simulink library "inp_lib"  (Simulink 7.4)
settings: Solver=ode45  StartTime=0.0  StopTime=10.0  RelTol=1e-3
settings Model: Creator=gephn  LastModifiedBy=wuqnj

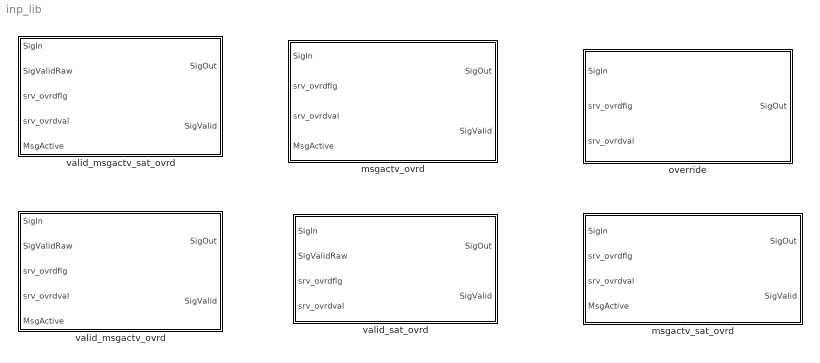
== system inp_lib ==
  msgactv_ovrd : Subsystem  mask{cal_ovrdflg=0, cal_ovrdval=0, default=0}
      mask prompts: cal_ovrdflg "Override Flag"; cal_ovrdval "Override Value"; default "Default Value"
  msgactv_sat_ovrd : Subsystem  mask{cal_ovrdflg=0, cal_ovrdval=0, default=0, hi=0, lo=0}
      mask prompts: cal_ovrdflg "Override Flag"; cal_ovrdval "Override Value"; default "Default Value"; hi "Range High"; lo "Range Low"
  override : Subsystem  mask{cal_ovrdflg=0, cal_ovrdval=0}
      mask prompts: cal_ovrdflg "Override Flag"; cal_ovrdval "Override Value"
  valid_msgactv_ovrd : Subsystem  AncestorBlock=inp_lib/valid_msgactv_sat_ovrd  mask{cal_ovrdflg=0, cal_ovrdval=0, lim=1, inc=1, dec=1, default=0}
      mask prompts: cal_ovrdflg "Override Flag"; cal_ovrdval "Override Value"; lim "Debounce Limit"; inc "Debounce Increment"; dec "Debounce Decrement"; default "Default Value"
  valid_msgactv_sat_ovrd : Subsystem  mask{cal_ovrdflg=0, cal_ovrdval=0, lim=1, inc=1, dec=1, default=0, hi=1, lo=0}
      mask prompts: cal_ovrdflg "Override Flag"; cal_ovrdval "Override Value"; lim "Debounce Limit"; inc "Debounce Increment"; dec "Debounce Decrement"; default "Default Value"; hi "Range High"; lo "Range Low"
  valid_sat_ovrd : Subsystem  mask{cal_ovrdflg=0, cal_ovrdval=0, lim=1, inc=1, dec=1, default=0, hi=1, lo=0}
      mask prompts: cal_ovrdflg "Override Flag"; cal_ovrdval "Override Value"; lim "Debounce Limit"; inc "Debounce Increment"; dec "Debounce Decrement"; default "Default Value"; hi "Range High"; lo "Range Low"

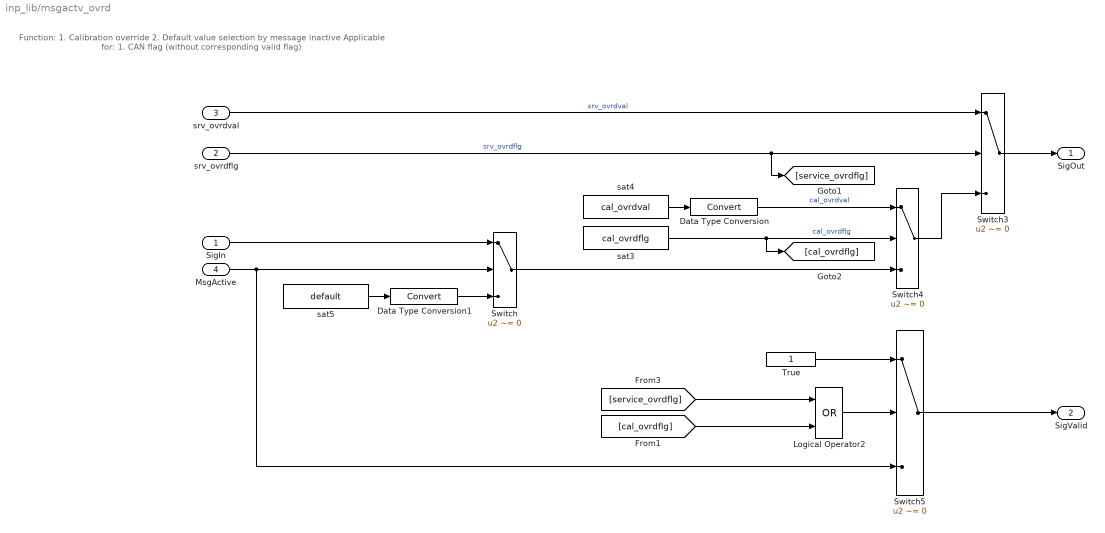
== system inp_lib/msgactv_ovrd ==
  note: Function:
      | 1. Calibration override
      | 2. Default value selection by message inactive
      | Applicable for:
      | 1. CAN flag  (without corresponding valid flag)
  SigIn : Inport  OutDataType=fixdt(1, 16)  OutScaling=2^0
  srv_ovrdflg : Inport  Port=2  OutDataType=fixdt(1, 16)  OutScaling=2^0
  srv_ovrdval : Inport  Port=3  OutDataType=fixdt(1, 16)  OutScaling=2^0
  MsgActive : Inport  Port=4  OutDataType=fixdt(1, 16)  OutScaling=2^0
  Data Type Conversion : DataTypeConversion  OutDataType=fixdt(1, 16)  OutScaling=2^0
  Data Type Conversion1 : DataTypeConversion  OutDataType=fixdt(1, 16)  OutScaling=2^0
  Logical Operator2 : Logic  Operator=OR  AllPortsSameDT=off  OutDataTypeMode=boolean  OutDataTypeStr=boolean
  Switch : Switch  Criteria=u2 ~= 0  OutDataType=fixdt(1, 16)  OutScaling=2^0
  Switch3 : Switch  Criteria=u2 ~= 0  Threshold=0.5  OutDataType=sfix(16)  OutScaling=2^0
  Switch4 : Switch  Criteria=u2 ~= 0  Threshold=0.5  OutDataType=sfix(16)  OutScaling=2^0
  Switch5 : Switch  Criteria=u2 ~= 0  Threshold=0.5  OutDataType=sfix(16)  OutScaling=2^0
  True : Constant  OutDataTypeMode=boolean  OutDataType=sfix(16)  OutScaling=2^0  OutDataTypeStr=boolean
  sat3 : Constant  Value=cal_ovrdflg  OutDataTypeMode=boolean  OutDataType=sfix(16)  OutScaling=2^0  OutDataTypeStr=boolean
  sat4 : Constant  Value=cal_ovrdval  OutDataType=sfix(16)  OutScaling=2^0  OutDataTypeStr=Inherit: Inherit via back propagation
  sat5 : Constant  Value=default  OutDataType=sfix(16)  OutScaling=2^0  OutDataTypeStr=Inherit: Inherit via back propagation
  SigOut : Outport  OutDataType=fixdt(1, 16)  OutScaling=2^0
  SigValid : Outport  Port=2  OutDataType=fixdt(1, 16)  OutScaling=2^0
  wires:
  sat4/1 -> Data Type Conversion/1
  SigIn/1 -> Switch/1
  MsgActive/1 -> Switch5/3, Switch/2
  sat5/1 -> Data Type Conversion1/1
  Data Type Conversion1/1 -> Switch/3
  [cal_ovrdflg] -> Logical Operator2/2
  [service_ovrdflg] -> Logical Operator2/1
  Switch3/1 -> SigOut/1
  srv_ovrdflg/1 -> [service_ovrdflg], Switch3/2  "srv_ovrdflg"
  sat3/1 -> [cal_ovrdflg], Switch4/2  "cal_ovrdflg"
  srv_ovrdval/1 -> Switch3/1  "srv_ovrdval"
  Data Type Conversion/1 -> Switch4/1  "cal_ovrdval"
  Switch4/1 -> Switch3/3
  Logical Operator2/1 -> Switch5/2
  True/1 -> Switch5/1
  Switch5/1 -> SigValid/1
  Switch/1 -> Switch4/3

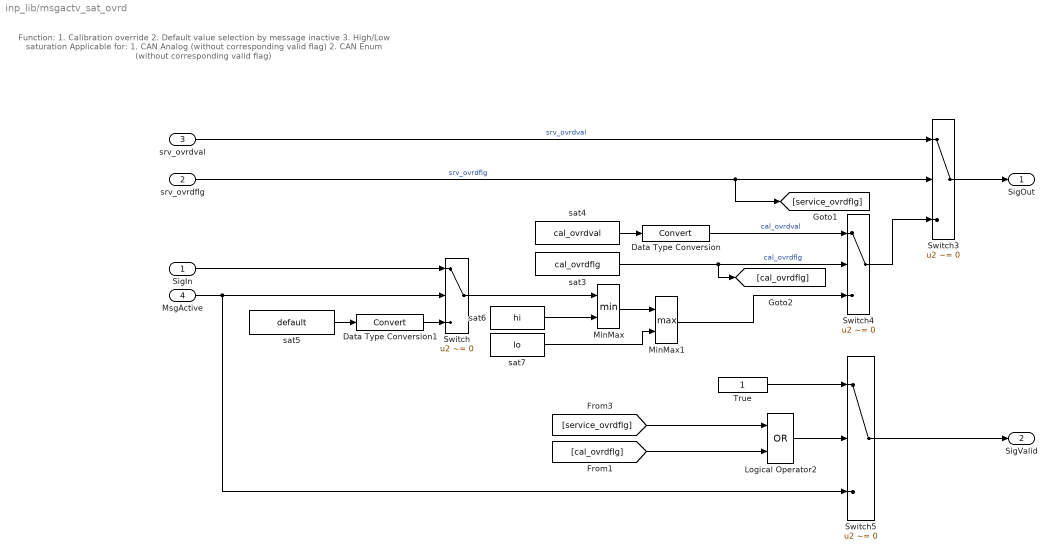
== system inp_lib/msgactv_sat_ovrd ==
  note: Function:
      | 1. Calibration override
      | 2. Default value selection by message inactive
      | 3. High/Low saturation
      | Applicable for:
      | 1. CAN Analog (without corresponding valid flag)
      | 2. CAN Enum (without corresponding valid flag)
  SigIn : Inport  OutDataType=fixdt(1, 16)  OutScaling=2^0
  srv_ovrdflg : Inport  Port=2  OutDataType=fixdt(1, 16)  OutScaling=2^0
  srv_ovrdval : Inport  Port=3  OutDataType=fixdt(1, 16)  OutScaling=2^0
  MsgActive : Inport  Port=4  OutDataType=fixdt(1, 16)  OutScaling=2^0
  Data Type Conversion : DataTypeConversion  OutDataType=fixdt(1, 16)  OutScaling=2^0
  Data Type Conversion1 : DataTypeConversion  OutDataType=fixdt(1, 16)  OutScaling=2^0
  Logical Operator2 : Logic  Operator=OR  AllPortsSameDT=off  OutDataTypeMode=boolean  OutDataTypeStr=boolean
  MinMax : MinMax  Inputs=2  OutDataType=fixdt(1, 16)  OutScaling=2^0
  MinMax1 : MinMax  Function=max  Inputs=2  OutDataType=fixdt(1, 16)  OutScaling=2^0
  Switch : Switch  Criteria=u2 ~= 0  OutDataType=fixdt(1, 16)  OutScaling=2^0
  Switch3 : Switch  Criteria=u2 ~= 0  Threshold=0.5  OutDataType=sfix(16)  OutScaling=2^0
  Switch4 : Switch  Criteria=u2 ~= 0  Threshold=0.5  OutDataType=sfix(16)  OutScaling=2^0
  Switch5 : Switch  Criteria=u2 ~= 0  Threshold=0.5  OutDataType=sfix(16)  OutScaling=2^0
  True : Constant  OutDataTypeMode=boolean  OutDataType=sfix(16)  OutScaling=2^0  OutDataTypeStr=boolean
  sat3 : Constant  Value=cal_ovrdflg  OutDataTypeMode=boolean  OutDataType=sfix(16)  OutScaling=2^0  OutDataTypeStr=boolean
  sat4 : Constant  Value=cal_ovrdval  OutDataType=sfix(16)  OutScaling=2^0  OutDataTypeStr=Inherit: Inherit via back propagation
  sat5 : Constant  Value=default  OutDataType=sfix(16)  OutScaling=2^0  OutDataTypeStr=Inherit: Inherit via back propagation
  sat6 : Constant  Value=hi  OutDataType=sfix(16)  OutScaling=2^0  OutDataTypeStr=Inherit: Inherit via back propagation
  sat7 : Constant  Value=lo  OutDataType=sfix(16)  OutScaling=2^0  OutDataTypeStr=Inherit: Inherit via back propagation
  SigOut : Outport  OutDataType=fixdt(1, 16)  OutScaling=2^0
  SigValid : Outport  Port=2  OutDataType=fixdt(1, 16)  OutScaling=2^0
  wires:
  Switch5/1 -> SigValid/1
  True/1 -> Switch5/1
  Logical Operator2/1 -> Switch5/2
  Switch4/1 -> Switch3/3
  Data Type Conversion/1 -> Switch4/1  "cal_ovrdval"
  srv_ovrdval/1 -> Switch3/1  "srv_ovrdval"
  sat3/1 -> Switch4/2, [cal_ovrdflg]  "cal_ovrdflg"
  srv_ovrdflg/1 -> Switch3/2, [service_ovrdflg]  "srv_ovrdflg"
  Switch3/1 -> SigOut/1
  [service_ovrdflg] -> Logical Operator2/1
  [cal_ovrdflg] -> Logical Operator2/2
  Data Type Conversion1/1 -> Switch/3
  sat5/1 -> Data Type Conversion1/1
  MsgActive/1 -> Switch/2, Switch5/3
  SigIn/1 -> Switch/1
  sat4/1 -> Data Type Conversion/1
  MinMax/1 -> MinMax1/1
  sat7/1 -> MinMax1/2
  sat6/1 -> MinMax/2
  Switch/1 -> MinMax/1
  MinMax1/1 -> Switch4/3

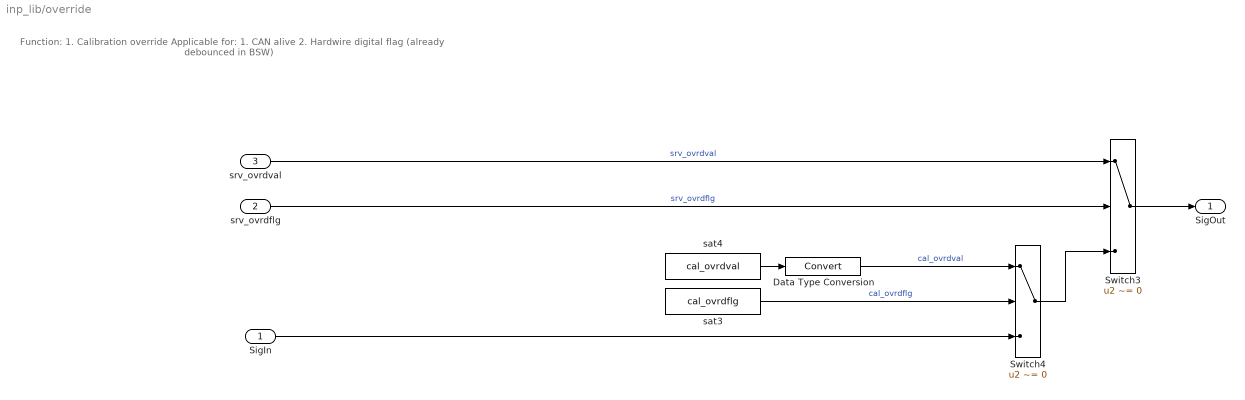
== system inp_lib/override ==
  note: Function:
      | 1. Calibration override
      | Applicable for:
      | 1. CAN alive
      | 2. Hardwire digital flag (already debounced in BSW)
  SigIn : Inport  OutDataType=fixdt(1, 16)  OutScaling=2^0
  srv_ovrdflg : Inport  Port=2  OutDataType=fixdt(1, 16)  OutScaling=2^0
  srv_ovrdval : Inport  Port=3  OutDataType=fixdt(1, 16)  OutScaling=2^0
  Data Type Conversion : DataTypeConversion  OutDataType=fixdt(1, 16)  OutScaling=2^0
  Switch3 : Switch  Criteria=u2 ~= 0  Threshold=0.5  OutDataType=sfix(16)  OutScaling=2^0
  Switch4 : Switch  Criteria=u2 ~= 0  Threshold=0.5  OutDataType=sfix(16)  OutScaling=2^0
  sat3 : Constant  Value=cal_ovrdflg  OutDataTypeMode=boolean  OutDataType=sfix(16)  OutScaling=2^0  OutDataTypeStr=boolean
  sat4 : Constant  Value=cal_ovrdval  OutDataType=sfix(16)  OutScaling=2^0  OutDataTypeStr=Inherit: Inherit via back propagation
  SigOut : Outport  OutDataType=fixdt(1, 16)  OutScaling=2^0
  wires:
  Switch4/1 -> Switch3/3
  Data Type Conversion/1 -> Switch4/1  "cal_ovrdval"
  srv_ovrdval/1 -> Switch3/1  "srv_ovrdval"
  sat3/1 -> Switch4/2  "cal_ovrdflg"
  srv_ovrdflg/1 -> Switch3/2  "srv_ovrdflg"
  Switch3/1 -> SigOut/1
  SigIn/1 -> Switch4/3
  sat4/1 -> Data Type Conversion/1

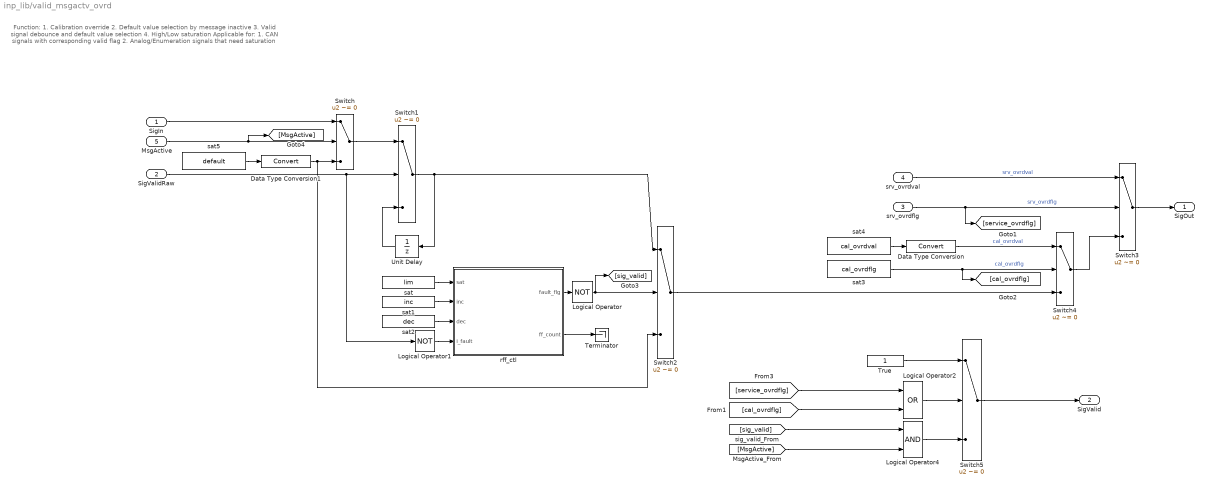
== system inp_lib/valid_msgactv_ovrd ==
  note: Function:
      | 1. Calibration override
      | 2. Default value selection by message inactive
      | 3. Valid signal debounce and default value selection
      | 4. High/Low saturation
      | Applicable for:
      | 1. CAN signals with corresponding valid flag
      | 2. Analog/Enumeration signals that need saturation
  SigIn : Inport  OutDataType=fixdt(1, 16)  OutScaling=2^0
  SigValidRaw : Inport  Port=2  OutDataType=fixdt(1, 16)  OutScaling=2^0
  srv_ovrdflg : Inport  Port=3  OutDataType=fixdt(1, 16)  OutScaling=2^0
  srv_ovrdval : Inport  Port=4  OutDataType=fixdt(1, 16)  OutScaling=2^0
  MsgActive : Inport  Port=5  OutDataType=fixdt(1, 16)  OutScaling=2^0
  Data Type Conversion : DataTypeConversion  OutDataType=fixdt(1, 16)  OutScaling=2^0
  Data Type Conversion1 : DataTypeConversion  OutDataType=fixdt(1, 16)  OutScaling=2^0
  Logical Operator : Logic  Operator=NOT  Inputs=1  AllPortsSameDT=off  OutDataTypeMode=boolean  LogicDataType=fixdt(0, 8)  OutDataTypeStr=boolean
  Logical Operator1 : Logic  Operator=NOT  Inputs=1  AllPortsSameDT=off  OutDataTypeMode=boolean  LogicDataType=fixdt(0, 8)  OutDataTypeStr=boolean
  Logical Operator2 : Logic  Operator=OR  AllPortsSameDT=off  OutDataTypeMode=boolean  OutDataTypeStr=boolean
  Logical Operator4 : Logic  AllPortsSameDT=off  OutDataTypeMode=boolean  OutDataTypeStr=boolean
  Switch : Switch  Criteria=u2 ~= 0  OutDataType=fixdt(1, 16)  OutScaling=2^0
  Switch1 : Switch  Criteria=u2 ~= 0  OutDataType=fixdt(1, 16)  OutScaling=2^0
  Switch2 : Switch  Criteria=u2 ~= 0  OutDataType=fixdt(1, 16)  OutScaling=2^0
  Switch3 : Switch  Criteria=u2 ~= 0  Threshold=0.5  OutDataType=sfix(16)  OutScaling=2^0
  Switch4 : Switch  Criteria=u2 ~= 0  Threshold=0.5  OutDataType=sfix(16)  OutScaling=2^0
  Switch5 : Switch  Criteria=u2 ~= 0  Threshold=0.5  OutDataType=sfix(16)  OutScaling=2^0
  Terminator : Terminator
  True : Constant  OutDataTypeMode=boolean  OutDataType=sfix(16)  OutScaling=2^0  OutDataTypeStr=boolean
  Unit Delay : UnitDelay  SampleTime=-1
      settings: AttributesFormatString=Init: %<X0>
  rff_ctl : Stateflow chart
  sat : Constant  Value=lim  OutDataTypeMode=uint8  OutDataType=sfix(16)  OutScaling=2^0  OutDataTypeStr=uint8
  sat1 : Constant  Value=inc  OutDataTypeMode=uint8  OutDataType=sfix(16)  OutScaling=2^0  OutDataTypeStr=uint8
  sat2 : Constant  Value=dec  OutDataTypeMode=uint8  OutDataType=sfix(16)  OutScaling=2^0  OutDataTypeStr=uint8
  sat3 : Constant  Value=cal_ovrdflg  OutDataTypeMode=boolean  OutDataType=sfix(16)  OutScaling=2^0  OutDataTypeStr=boolean
  sat4 : Constant  Value=cal_ovrdval  OutDataType=sfix(16)  OutScaling=2^0  OutDataTypeStr=Inherit: Inherit via back propagation
  sat5 : Constant  Value=default  OutDataType=sfix(16)  OutScaling=2^0  OutDataTypeStr=Inherit: Inherit via back propagation
  SigOut : Outport  OutDataType=fixdt(1, 16)  OutScaling=2^0
  SigValid : Outport  Port=2  OutDataType=fixdt(1, 16)  OutScaling=2^0
  wires:
  sat4/1 -> Data Type Conversion/1
  SigIn/1 -> Switch/1
  MsgActive/1 -> Switch/2, [MsgActive]
  sat5/1 -> Data Type Conversion1/1
  Switch/1 -> Switch1/1
  sat/1 -> rff_ctl/1(sat)
  sat1/1 -> rff_ctl/2(inc)
  sat2/1 -> rff_ctl/3(dec)
  rff_ctl/1(fault_flg) -> Logical Operator/1
  rff_ctl/2(ff_count) -> Terminator/1
  Data Type Conversion1/1 -> Switch/3, Switch2/3
  Switch1/1 -> Unit Delay/1, Switch2/1
  Unit Delay/1 -> Switch1/3
  Logical Operator1/1 -> rff_ctl/4(i_fault)
  SigValidRaw/1 -> Switch1/2, Logical Operator1/1
  [cal_ovrdflg] -> Logical Operator2/2
  [service_ovrdflg] -> Logical Operator2/1
  Switch3/1 -> SigOut/1
  srv_ovrdflg/1 -> [service_ovrdflg], Switch3/2  "srv_ovrdflg"
  sat3/1 -> [cal_ovrdflg], Switch4/2  "cal_ovrdflg"
  srv_ovrdval/1 -> Switch3/1  "srv_ovrdval"
  Data Type Conversion/1 -> Switch4/1  "cal_ovrdval"
  Switch4/1 -> Switch3/3
  Logical Operator2/1 -> Switch5/2
  True/1 -> Switch5/1
  Switch5/1 -> SigValid/1
  Logical Operator/1 -> Switch2/2, [sig_valid]
  [MsgActive] -> Logical Operator4/2
  [sig_valid] -> Logical Operator4/1
  Logical Operator4/1 -> Switch5/3
  Switch2/1 -> Switch4/3

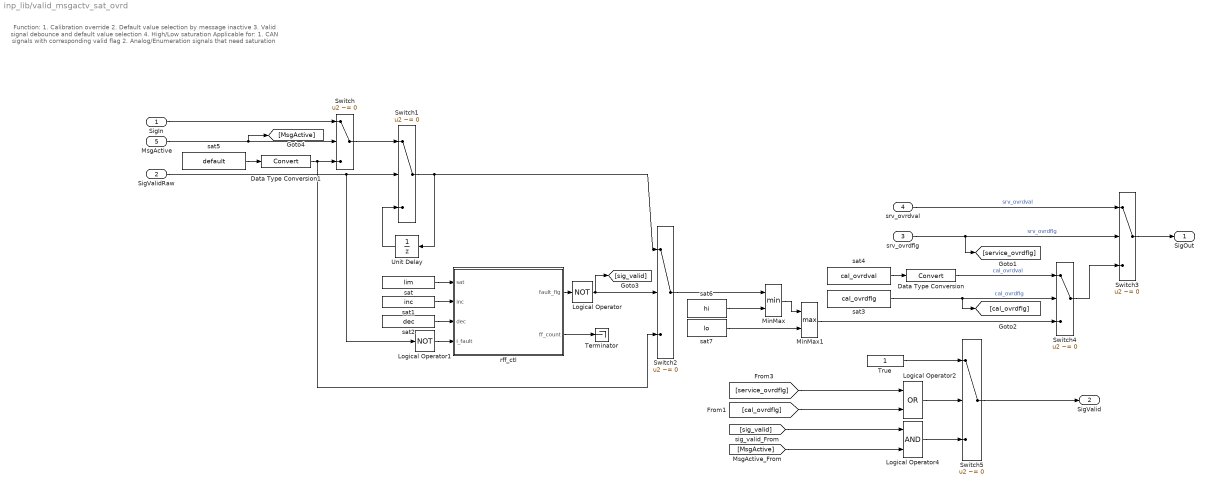
== system inp_lib/valid_msgactv_sat_ovrd ==
  note: Function:
      | 1. Calibration override
      | 2. Default value selection by message inactive
      | 3. Valid signal debounce and default value selection
      | 4. High/Low saturation
      | Applicable for:
      | 1. CAN signals with corresponding valid flag
      | 2. Analog/Enumeration signals that need saturation
  SigIn : Inport  OutDataType=fixdt(1, 16)  OutScaling=2^0
  SigValidRaw : Inport  Port=2  OutDataType=fixdt(1, 16)  OutScaling=2^0
  srv_ovrdflg : Inport  Port=3  OutDataType=fixdt(1, 16)  OutScaling=2^0
  srv_ovrdval : Inport  Port=4  OutDataType=fixdt(1, 16)  OutScaling=2^0
  MsgActive : Inport  Port=5  OutDataType=fixdt(1, 16)  OutScaling=2^0
  Data Type Conversion : DataTypeConversion  OutDataType=fixdt(1, 16)  OutScaling=2^0
  Data Type Conversion1 : DataTypeConversion  OutDataType=fixdt(1, 16)  OutScaling=2^0
  Logical Operator : Logic  Operator=NOT  Inputs=1  AllPortsSameDT=off  OutDataTypeMode=boolean  LogicDataType=fixdt(0, 8)  OutDataTypeStr=boolean
  Logical Operator1 : Logic  Operator=NOT  Inputs=1  AllPortsSameDT=off  OutDataTypeMode=boolean  LogicDataType=fixdt(0, 8)  OutDataTypeStr=boolean
  Logical Operator2 : Logic  Operator=OR  AllPortsSameDT=off  OutDataTypeMode=boolean  OutDataTypeStr=boolean
  Logical Operator4 : Logic  AllPortsSameDT=off  OutDataTypeMode=boolean  OutDataTypeStr=boolean
  MinMax : MinMax  Inputs=2  OutDataType=fixdt(1, 16)  OutScaling=2^0
  MinMax1 : MinMax  Function=max  Inputs=2  OutDataType=fixdt(1, 16)  OutScaling=2^0
  Switch : Switch  Criteria=u2 ~= 0  OutDataType=fixdt(1, 16)  OutScaling=2^0
  Switch1 : Switch  Criteria=u2 ~= 0  OutDataType=fixdt(1, 16)  OutScaling=2^0
  Switch2 : Switch  Criteria=u2 ~= 0  OutDataType=fixdt(1, 16)  OutScaling=2^0
  Switch3 : Switch  Criteria=u2 ~= 0  Threshold=0.5  OutDataType=sfix(16)  OutScaling=2^0
  Switch4 : Switch  Criteria=u2 ~= 0  Threshold=0.5  OutDataType=sfix(16)  OutScaling=2^0
  Switch5 : Switch  Criteria=u2 ~= 0  Threshold=0.5  OutDataType=sfix(16)  OutScaling=2^0
  Terminator : Terminator
  True : Constant  OutDataTypeMode=boolean  OutDataType=sfix(16)  OutScaling=2^0  OutDataTypeStr=boolean
  Unit Delay : UnitDelay  SampleTime=-1
      settings: AttributesFormatString=Init: %<X0>
  rff_ctl : Stateflow chart
  sat : Constant  Value=lim  OutDataTypeMode=uint8  OutDataType=sfix(16)  OutScaling=2^0  OutDataTypeStr=uint8
  sat1 : Constant  Value=inc  OutDataTypeMode=uint8  OutDataType=sfix(16)  OutScaling=2^0  OutDataTypeStr=uint8
  sat2 : Constant  Value=dec  OutDataTypeMode=uint8  OutDataType=sfix(16)  OutScaling=2^0  OutDataTypeStr=uint8
  sat3 : Constant  Value=cal_ovrdflg  OutDataTypeMode=boolean  OutDataType=sfix(16)  OutScaling=2^0  OutDataTypeStr=boolean
  sat4 : Constant  Value=cal_ovrdval  OutDataType=sfix(16)  OutScaling=2^0  OutDataTypeStr=Inherit: Inherit via back propagation
  sat5 : Constant  Value=default  OutDataType=sfix(16)  OutScaling=2^0  OutDataTypeStr=Inherit: Inherit via back propagation
  sat6 : Constant  Value=hi  OutDataType=sfix(16)  OutScaling=2^0  OutDataTypeStr=Inherit: Inherit via back propagation
  sat7 : Constant  Value=lo  OutDataType=sfix(16)  OutScaling=2^0  OutDataTypeStr=Inherit: Inherit via back propagation
  SigOut : Outport  OutDataType=fixdt(1, 16)  OutScaling=2^0
  SigValid : Outport  Port=2  OutDataType=fixdt(1, 16)  OutScaling=2^0
  wires:
  sat4/1 -> Data Type Conversion/1
  SigIn/1 -> Switch/1
  MsgActive/1 -> Switch/2, [MsgActive]
  sat5/1 -> Data Type Conversion1/1
  Switch/1 -> Switch1/1
  sat/1 -> rff_ctl/1(sat)
  sat1/1 -> rff_ctl/2(inc)
  sat2/1 -> rff_ctl/3(dec)
  rff_ctl/1(fault_flg) -> Logical Operator/1
  rff_ctl/2(ff_count) -> Terminator/1
  Data Type Conversion1/1 -> Switch/3, Switch2/3
  Switch1/1 -> Unit Delay/1, Switch2/1
  Unit Delay/1 -> Switch1/3
  Logical Operator1/1 -> rff_ctl/4(i_fault)
  SigValidRaw/1 -> Switch1/2, Logical Operator1/1
  [cal_ovrdflg] -> Logical Operator2/2
  [service_ovrdflg] -> Logical Operator2/1
  Switch3/1 -> SigOut/1
  srv_ovrdflg/1 -> [service_ovrdflg], Switch3/2  "srv_ovrdflg"
  sat3/1 -> [cal_ovrdflg], Switch4/2  "cal_ovrdflg"
  srv_ovrdval/1 -> Switch3/1  "srv_ovrdval"
  Data Type Conversion/1 -> Switch4/1  "cal_ovrdval"
  Switch4/1 -> Switch3/3
  Logical Operator2/1 -> Switch5/2
  True/1 -> Switch5/1
  Switch5/1 -> SigValid/1
  Logical Operator/1 -> Switch2/2, [sig_valid]
  [MsgActive] -> Logical Operator4/2
  [sig_valid] -> Logical Operator4/1
  Logical Operator4/1 -> Switch5/3
  MinMax/1 -> MinMax1/1
  sat7/1 -> MinMax1/2
  sat6/1 -> MinMax/2
  Switch2/1 -> MinMax/1
  MinMax1/1 -> Switch4/3

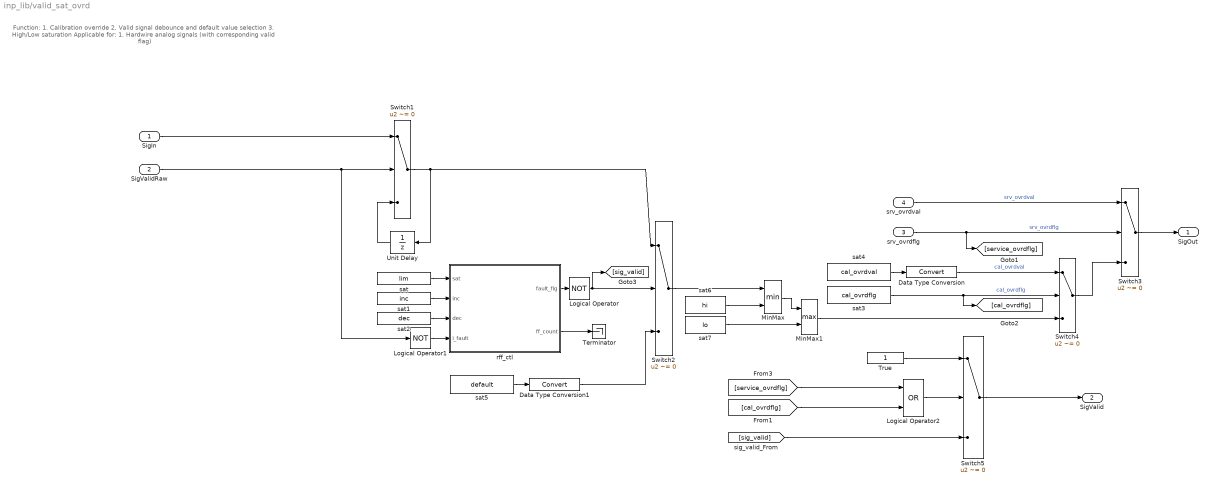
== system inp_lib/valid_sat_ovrd ==
  note: Function:
      | 1. Calibration override
      | 2. Valid signal debounce and default value selection
      | 3. High/Low saturation
      | Applicable for:
      | 1. Hardwire analog signals (with corresponding valid flag)
  SigIn : Inport  OutDataType=fixdt(1, 16)  OutScaling=2^0
  SigValidRaw : Inport  Port=2  OutDataType=fixdt(1, 16)  OutScaling=2^0
  srv_ovrdflg : Inport  Port=3  OutDataType=fixdt(1, 16)  OutScaling=2^0
  srv_ovrdval : Inport  Port=4  OutDataType=fixdt(1, 16)  OutScaling=2^0
  Data Type Conversion : DataTypeConversion  OutDataType=fixdt(1, 16)  OutScaling=2^0
  Data Type Conversion1 : DataTypeConversion  OutDataType=fixdt(1, 16)  OutScaling=2^0
  Logical Operator : Logic  Operator=NOT  Inputs=1  AllPortsSameDT=off  OutDataTypeMode=boolean  LogicDataType=fixdt(0, 8)  OutDataTypeStr=boolean
  Logical Operator1 : Logic  Operator=NOT  Inputs=1  AllPortsSameDT=off  OutDataTypeMode=boolean  LogicDataType=fixdt(0, 8)  OutDataTypeStr=boolean
  Logical Operator2 : Logic  Operator=OR  AllPortsSameDT=off  OutDataTypeMode=boolean  OutDataTypeStr=boolean
  MinMax : MinMax  Inputs=2  OutDataType=fixdt(1, 16)  OutScaling=2^0
  MinMax1 : MinMax  Function=max  Inputs=2  OutDataType=fixdt(1, 16)  OutScaling=2^0
  Switch1 : Switch  Criteria=u2 ~= 0  OutDataType=fixdt(1, 16)  OutScaling=2^0
  Switch2 : Switch  Criteria=u2 ~= 0  OutDataType=fixdt(1, 16)  OutScaling=2^0
  Switch3 : Switch  Criteria=u2 ~= 0  Threshold=0.5  OutDataType=sfix(16)  OutScaling=2^0
  Switch4 : Switch  Criteria=u2 ~= 0  Threshold=0.5  OutDataType=sfix(16)  OutScaling=2^0
  Switch5 : Switch  Criteria=u2 ~= 0  Threshold=0.5  OutDataType=sfix(16)  OutScaling=2^0
  Terminator : Terminator
  True : Constant  OutDataTypeMode=boolean  OutDataType=sfix(16)  OutScaling=2^0  OutDataTypeStr=boolean
  Unit Delay : UnitDelay  SampleTime=-1
      settings: AttributesFormatString=Init: %<X0>
  rff_ctl : Stateflow chart
  sat : Constant  Value=lim  OutDataTypeMode=uint8  OutDataType=sfix(16)  OutScaling=2^0  OutDataTypeStr=uint8
  sat1 : Constant  Value=inc  OutDataTypeMode=uint8  OutDataType=sfix(16)  OutScaling=2^0  OutDataTypeStr=uint8
  sat2 : Constant  Value=dec  OutDataTypeMode=uint8  OutDataType=sfix(16)  OutScaling=2^0  OutDataTypeStr=uint8
  sat3 : Constant  Value=cal_ovrdflg  OutDataTypeMode=boolean  OutDataType=sfix(16)  OutScaling=2^0  OutDataTypeStr=boolean
  sat4 : Constant  Value=cal_ovrdval  OutDataType=sfix(16)  OutScaling=2^0  OutDataTypeStr=Inherit: Inherit via back propagation
  sat5 : Constant  Value=default  OutDataType=sfix(16)  OutScaling=2^0  OutDataTypeStr=Inherit: Inherit via back propagation
  sat6 : Constant  Value=hi  OutDataType=sfix(16)  OutScaling=2^0  OutDataTypeStr=Inherit: Inherit via back propagation
  sat7 : Constant  Value=lo  OutDataType=sfix(16)  OutScaling=2^0  OutDataTypeStr=Inherit: Inherit via back propagation
  SigOut : Outport  OutDataType=fixdt(1, 16)  OutScaling=2^0
  SigValid : Outport  Port=2  OutDataType=fixdt(1, 16)  OutScaling=2^0
  wires:
  MinMax1/1 -> Switch4/3
  Switch2/1 -> MinMax/1
  sat6/1 -> MinMax/2
  sat7/1 -> MinMax1/2
  MinMax/1 -> MinMax1/1
  [sig_valid] -> Switch5/3
  Logical Operator/1 -> [sig_valid], Switch2/2
  Switch5/1 -> SigValid/1
  True/1 -> Switch5/1
  Logical Operator2/1 -> Switch5/2
  Switch4/1 -> Switch3/3
  Data Type Conversion/1 -> Switch4/1  "cal_ovrdval"
  srv_ovrdval/1 -> Switch3/1  "srv_ovrdval"
  sat3/1 -> Switch4/2, [cal_ovrdflg]  "cal_ovrdflg"
  srv_ovrdflg/1 -> Switch3/2, [service_ovrdflg]  "srv_ovrdflg"
  Switch3/1 -> SigOut/1
  [service_ovrdflg] -> Logical Operator2/1
  [cal_ovrdflg] -> Logical Operator2/2
  SigValidRaw/1 -> Logical Operator1/1, Switch1/2
  Logical Operator1/1 -> rff_ctl/4(i_fault)
  Unit Delay/1 -> Switch1/3
  Switch1/1 -> Switch2/1, Unit Delay/1
  Data Type Conversion1/1 -> Switch2/3
  rff_ctl/2(ff_count) -> Terminator/1
  rff_ctl/1(fault_flg) -> Logical Operator/1
  sat2/1 -> rff_ctl/3(dec)
  sat1/1 -> rff_ctl/2(inc)
  sat/1 -> rff_ctl/1(sat)
  sat5/1 -> Data Type Conversion1/1
  SigIn/1 -> Switch1/1
  sat4/1 -> Data Type Conversion/1

== stateflow chart valid_sat_ovrd/rff_ctl ==
  (default) -> (junction 3)
  (junction 3) -> (junction 7) [order 2] : {count-=dec;}
  (junction 3) -> (junction 7) [order 1] : [i_fault]
      | {count+=inc;}
  (junction 4) -> (junction 5) [order 1] : [count>=sat]
      | {count=sat;
      | fault_flg=1;}
  (junction 4) -> (junction 5) [order 2] : [count<=0]
      | {count=0;
      | fault_flg=0;}
  (junction 4) -> (junction 5) [order 3]
  (junction 5) -> (junction 6) : {ff_count = count;}
  (junction 7) -> (junction 4)
  data: sat input uint8; inc input uint8; dec input uint8; i_fault input boolean; fault_flg output boolean =0; ff_count output uint8; count local int16

== stateflow chart valid_msgactv_ovrd/rff_ctl ==
  (default) -> (junction 25)
  (junction 25) -> (junction 29) [order 2] : {count-=dec;}
  (junction 25) -> (junction 29) [order 1] : [i_fault]
      | {count+=inc;}
  (junction 26) -> (junction 27) [order 1] : [count>=sat]
      | {count=sat;
      | fault_flg=1;}
  (junction 26) -> (junction 27) [order 2] : [count<=0]
      | {count=0;
      | fault_flg=0;}
  (junction 26) -> (junction 27) [order 3]
  (junction 27) -> (junction 28) : {ff_count = count;}
  (junction 29) -> (junction 26)
  data: sat input uint8; inc input uint8; dec input uint8; i_fault input boolean; fault_flg output boolean =0; ff_count output uint8; count local int16

== stateflow chart valid_msgactv_sat_ovrd/rff_ctl ==
  (default) -> (junction 47)
  (junction 47) -> (junction 51) [order 2] : {count-=dec;}
  (junction 47) -> (junction 51) [order 1] : [i_fault]
      | {count+=inc;}
  (junction 48) -> (junction 49) [order 1] : [count>=sat]
      | {count=sat;
      | fault_flg=1;}
  (junction 48) -> (junction 49) [order 2] : [count<=0]
      | {count=0;
      | fault_flg=0;}
  (junction 48) -> (junction 49) [order 3]
  (junction 49) -> (junction 50) : {ff_count = count;}
  (junction 51) -> (junction 48)
  data: sat input uint8; inc input uint8; dec input uint8; i_fault input boolean; fault_flg output boolean =0; ff_count output uint8; count local int16
